simulink model "sixth_harmonic_report"  (R2013a)
settings: Solver=ode4  StartTime=0.0  StopTime=0.5  FixedStep=Ts  RelTol=1e-3
values from neighbouring files (symbols this model uses):
  Cdc = 200e-6    (= 0.0002)    [immd_design_elen.m]    (also in immd_efficiency.m = 5e-05; immd_simulation_base.m = 5e-05; sixth_harmonic_report.m = 0.003)
  Ldc = 1e-3    (= 0.001)    [sixth_harmonic_report.m]
  Lload = Xload/wout_fund    [acemp_sixth.m]    (also in immd_base_varyingmod.m = Xload/wout; immd_design_elen.m = Xload/wout; immd_efficiency.m = Xload/wout; immd_simulation_base.m = Xload/wout)
  Rload = Zload*pf    [acemp_sixth.m]    (also in immd_base_varyingmod.m; immd_design_elen.m; immd_efficiency.m; immd_simulation_base.m)
  Ts = 1e-6    (= 1e-06)    [acemp_sixth.m]    (also in immd_base_varyingmod.m = 1e-05; immd_design_elen.m; immd_efficiency.m; immd_simulation_base.m)
  Vsrms = 230    [sixth_harmonic_report.m]
libraries: powerlib x27, powerlib_meascontrol x27
settings Model: Creator=ugurm  LastModifiedBy=ugurm

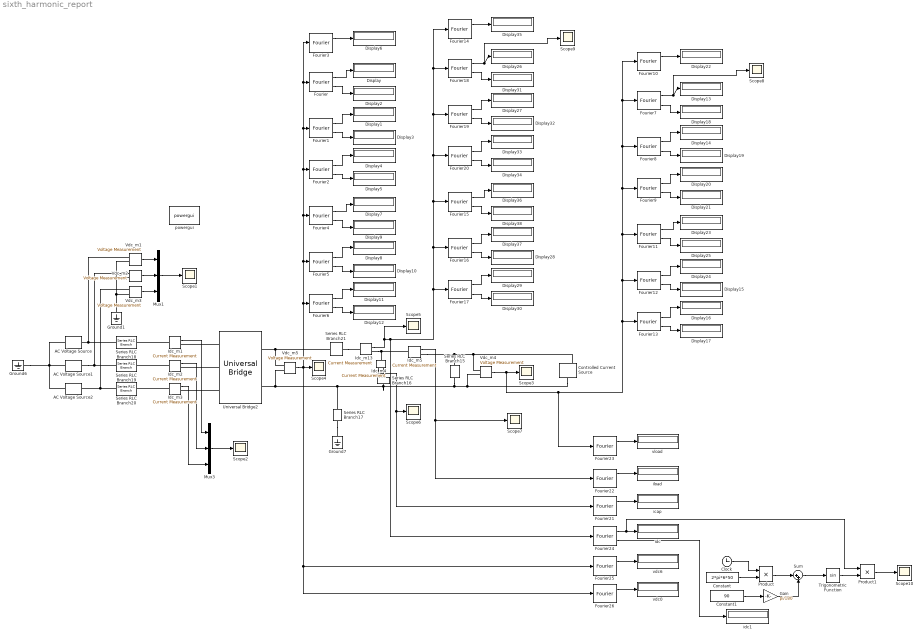
== system sixth_harmonic_report ==
  AC Voltage Source : powerlib/Electrical Sources/AC Voltage Source  Amplitude=Vsrms*sqrt(2)  Phase=0  Frequency=50  SampleTime=Ts  Measurements=None
  AC Voltage Source1 : powerlib/Electrical Sources/AC Voltage Source  Amplitude=Vsrms*sqrt(2)  Phase=-120  Frequency=50  SampleTime=Ts  Measurements=None
  AC Voltage Source2 : powerlib/Electrical Sources/AC Voltage Source  Amplitude=Vsrms*sqrt(2)  Phase=120  Frequency=50  SampleTime=Ts  Measurements=None
  Clock : Clock
  Constant : Constant  Value=2*pi*6*50
  Constant1 : Constant  Value=90
  Controlled Current Source : powerlib/Electrical Sources/Controlled Current Source  Initialize=on  Source_Type=AC  Amplitude=0  Phase=0  Frequency=0  Measurements=None
  Display{,1..38} (39 alike) : Display
  Fourier{,7,18,21..25} (8 alike) : powerlib_meascontrol/Measurements/Fourier  Freq=50  n=6  InInit=[0, 0]  Ts=0
  Fourier1 : powerlib_meascontrol/Measurements/Fourier  Freq=50  n=12  InInit=[0, 0]  Ts=0
  Fourier{3,10,14,26} (4 alike) : powerlib_meascontrol/Measurements/Fourier  Freq=50  n=0  InInit=[0, 0]  Ts=0
  Fourier11 : powerlib_meascontrol/Measurements/Fourier  Freq=50  n=24  InInit=[0, 0]  Ts=0
  Fourier12 : powerlib_meascontrol/Measurements/Fourier  Freq=50  n=30  InInit=[0, 0]  Ts=0
  Fourier13 : powerlib_meascontrol/Measurements/Fourier  Freq=50  n=36  InInit=[0, 0]  Ts=0
  Fourier15 : powerlib_meascontrol/Measurements/Fourier  Freq=50  n=24  InInit=[0, 0]  Ts=0
  Fourier16 : powerlib_meascontrol/Measurements/Fourier  Freq=50  n=30  InInit=[0, 0]  Ts=0
  Fourier17 : powerlib_meascontrol/Measurements/Fourier  Freq=50  n=36  InInit=[0, 0]  Ts=0
  Fourier19 : powerlib_meascontrol/Measurements/Fourier  Freq=50  n=12  InInit=[0, 0]  Ts=0
  Fourier2 : powerlib_meascontrol/Measurements/Fourier  Freq=50  n=18  InInit=[0, 0]  Ts=0
  Fourier20 : powerlib_meascontrol/Measurements/Fourier  Freq=50  n=18  InInit=[0, 0]  Ts=0
  Fourier4 : powerlib_meascontrol/Measurements/Fourier  Freq=50  n=24  InInit=[0, 0]  Ts=0
  Fourier5 : powerlib_meascontrol/Measurements/Fourier  Freq=50  n=30  InInit=[0, 0]  Ts=0
  Fourier6 : powerlib_meascontrol/Measurements/Fourier  Freq=50  n=36  InInit=[0, 0]  Ts=0
  Fourier8 : powerlib_meascontrol/Measurements/Fourier  Freq=50  n=12  InInit=[0, 0]  Ts=0
  Fourier9 : powerlib_meascontrol/Measurements/Fourier  Freq=50  n=18  InInit=[0, 0]  Ts=0
  Gain : Gain  Gain=pi/180
  Ground1 : powerlib/Elements/Ground  LConnTagsString=a
  Ground6 : powerlib/Elements/Ground  LConnTagsString=a
  Ground7 : powerlib/Elements/Ground  LConnTagsString=a
  Idc_m{1..5,13} (6 alike) : powerlib/Measurements/Current Measurement  PhasorSimulation=off  OutputType=Complex  PSBequivalent=0
  Mux1 : Mux  Inputs=3
  Mux3 : Mux  Inputs=3
  Product : Product
  Product1 : Product
  Scope{1..10} (10 alike) : Scope
      Scope1 settings: YMin=-1000  YMax=18000  SaveName=vabc
      Scope10 settings: YMin=-1  YMax=1  SaveName=iload1
      Scope2 settings: YMin=-1000  YMax=18000  SaveName=iabc
      Scope3 settings: YMin=-1000  YMax=18000  SaveName=vload
      Scope4 settings: YMin=-1000  YMax=18000  SaveName=vdc
      Scope5 settings: YMin=-1000  YMax=18000  SaveName=idc
      Scope6 settings: YMin=-1000  YMax=18000  SaveName=ic
      Scope7 settings: YMin=-1000  YMax=18000  SaveName=iload
      Scope8 settings: YMin=2.9  YMax=3.55  SaveName=vload1
      Scope9 settings: YMin=17.3  YMax=18.9  SaveName=vload2
  Series RLC Branch15 : powerlib/Elements/Series RLC Branch  LConnTagsString=__new0  RConnTagsString=__new0  BranchType=R  Resistance=Rload  Inductance=Lload  SetiL0=off  InitialCurrent=0  Capacitance=1e-6  Setx0=off  InitialVoltage=0  Measurements=None
  Series RLC Branch16 : powerlib/Elements/Series RLC Branch  LConnTagsString=__new0  RConnTagsString=__new0  BranchType=RC  Resistance=1e-9  Inductance=Lload  SetiL0=off  InitialCurrent=0  Capacitance=Cdc  Setx0=off  InitialVoltage=0  Measurements=None
  Series RLC Branch17 : powerlib/Elements/Series RLC Branch  LConnTagsString=__new0  RConnTagsString=__new0  BranchType=R  Resistance=1e12  Inductance=Lload  SetiL0=off  InitialCurrent=0  Capacitance=1e-6  Setx0=off  InitialVoltage=0  Measurements=None
  Series RLC Branch18 : powerlib/Elements/Series RLC Branch  LConnTagsString=__new0  RConnTagsString=__new0  BranchType=RL  Resistance=1e-6  Inductance=1e-9  SetiL0=off  InitialCurrent=0  Capacitance=100e-6  Setx0=off  InitialVoltage=0  Measurements=None
  Series RLC Branch19 : powerlib/Elements/Series RLC Branch  LConnTagsString=__new0  RConnTagsString=__new0  BranchType=RL  Resistance=1e-6  Inductance=1e-9  SetiL0=off  InitialCurrent=0  Capacitance=100e-6  Setx0=off  InitialVoltage=0  Measurements=None
  Series RLC Branch20 : powerlib/Elements/Series RLC Branch  LConnTagsString=__new0  RConnTagsString=__new0  BranchType=RL  Resistance=1e-6  Inductance=1e-9  SetiL0=off  InitialCurrent=0  Capacitance=100e-6  Setx0=off  InitialVoltage=0  Measurements=None
  Series RLC Branch21 : powerlib/Elements/Series RLC Branch  LConnTagsString=__new0  RConnTagsString=__new0  BranchType=RL  Resistance=1e-6  Inductance=Ldc  SetiL0=off  InitialCurrent=0  Capacitance=100e-6  Setx0=off  InitialVoltage=0  Measurements=None
  Sum : Sum  Inputs=|++
  Trigonometric Function : Trigonometry
  Universal Bridge2 : powerlib/Power Electronics/Universal Bridge  Arms=3  SnubberResistance=1e5  SnubberCapacitance=inf  Device=Diodes  Ron=1e-6  Lon=0  ForwardVoltages="[  0  0  ]"  ForwardVoltage=0  GTOparameters=[ 10e-6 , 20e-6 ]  IGBTparameters=[0,0]  Measurements=None  Measurements_2=None  converterType=Rectifier
  Vdc_m{1..5} (5 alike) : powerlib/Measurements/Voltage Measurement  PhasorSimulation=off  OutputType=Complex  PSBequivalent=0
  icap : Display
  idc : Display
  idc1 : Display
  iload : Display
  powergui : powerlib/powergui  Priority=1  SimulationMode=Discrete  SolverType=Tustin  SampleTime=Ts  frequency=60  SPID=off  DisableSnubberDevices=off  DisableRonSwitches=off  DisableVfSwitches=off  SwTol=0  Interpol=off  DisplayEquations=off  frequencyindice=0  Pbase=100e6  ErrMax=1e-4  Iterations=50  UnitsV=kV  UnitsW=MW  FunctionMessages=off  echomessages=off  HookPort=off  EnableUseOfTLC=off  x0status=blocks  RestoreLinks=warning  ResistiveCurrentMeasurement=off  Frange=[0:2:500]  Ylog=off  Xlog=on  ShowGrid=off  save=off  variable=ZData  structure=vdc  ZoomFFT=off  StartTime=0.1  cycles=10  DisplayStyle=6  fundamental=50  FreqAxis=off  MaxFrequency=1000  frequencyindicesteady=1  RmsSteady=1  display=off  Ts=0  methode=off
  vdc0 : Display
  vdc6 : Display
  vload : Display
  wires:
  Vdc_m1/1 -> Mux1/1
  Vdc_m2/1 -> Mux1/2
  Vdc_m3/1 -> Mux1/3
  Mux1/1 -> Scope1/1
  Mux3/1 -> Scope2/1
  Idc_m1/1 -> Mux3/1
  Idc_m2/1 -> Mux3/2
  Idc_m3/1 -> Mux3/3
  Fourier/1 -> Display/1
  Fourier1/1 -> Display1/1
  Fourier/2 -> Display2/1
  Fourier1/2 -> Display3/1
  Fourier2/1 -> Display4/1
  Fourier2/2 -> Display5/1
  Fourier3/1 -> Display6/1
  Fourier4/1 -> Display7/1
  Fourier5/1 -> Display8/1
  Fourier4/2 -> Display9/1
  Fourier5/2 -> Display10/1
  Fourier6/1 -> Display11/1
  Fourier6/2 -> Display12/1
  Vdc_m4/1 -> Scope3/1, Fourier23/1, Fourier12/1, Fourier11/1, Fourier10/1, Fourier7/1, Fourier8/1, Fourier9/1, Fourier13/1
  Fourier7/1 -> Scope8/1, Display13/1
  Fourier8/1 -> Display14/1
  Fourier7/2 -> Display18/1
  Fourier8/2 -> Display19/1
  Fourier9/1 -> Display20/1
  Fourier9/2 -> Display21/1
  Fourier10/1 -> Display22/1
  Fourier11/1 -> Display23/1
  Fourier12/1 -> Display24/1
  Fourier11/2 -> Display25/1
  Fourier12/2 -> Display15/1
  Fourier13/1 -> Display16/1
  Fourier13/2 -> Display17/1
  Fourier18/1 -> Scope9/1, Display26/1
  Fourier19/1 -> Display27/1
  Fourier18/2 -> Display31/1
  Fourier19/2 -> Display32/1
  Fourier20/1 -> Display33/1
  Fourier20/2 -> Display34/1
  Fourier14/1 -> Display35/1
  Fourier15/1 -> Display36/1
  Fourier16/1 -> Display37/1
  Fourier15/2 -> Display38/1
  Fourier16/2 -> Display28/1
  Fourier17/1 -> Display29/1
  Fourier17/2 -> Display30/1
  Idc_m5/1 -> Fourier22/1, Scope7/1
  Idc_m4/1 -> Fourier21/1, Scope6/1
  Fourier21/1 -> icap/1
  Fourier22/1 -> iload/1
  Fourier23/1 -> vload/1
  Idc_m13/1 -> Fourier24/1, Fourier16/1, Fourier15/1, Fourier14/1, Fourier18/1, Fourier19/1, Fourier20/1, Fourier17/1, Scope5/1
  Vdc_m5/1 -> Fourier6/1, Fourier5/1, Fourier4/1, Fourier2/1, Fourier1/1, Fourier3/1, Fourier/1, Fourier26/1, Fourier25/1, Scope4/1
  Fourier25/1 -> vdc6/1
  Fourier26/1 -> vdc0/1
  Fourier24/2 -> idc1/1
  Clock/1 -> Product/1
  Constant/1 -> Product/2
  Product/1 -> Sum/1
  Gain/1 -> Sum/2
  Constant1/1 -> Gain/1
  Sum/1 -> Trigonometric Function/1
  Trigonometric Function/1 -> Product1/2
  Product1/1 -> Scope10/1
  Fourier24/1 -> Product1/1, idc/1
  connections:
  Vdc_m4/LConn1 -- Controlled Current Source/LConn1 -- Series RLC Branch15/RConn1 -- Idc_m5/RConn1
  Vdc_m4/LConn2 -- Controlled Current Source/RConn1 -- Series RLC Branch17/LConn1 -- Vdc_m5/LConn2 -- Universal Bridge2/RConn2 -- Series RLC Branch16/RConn1 -- Series RLC Branch15/LConn1
  Series RLC Branch17/RConn1 -- Ground7/LConn1
  Series RLC Branch20/RConn1 -- Vdc_m3/LConn1 -- AC Voltage Source2/RConn1
  AC Voltage Source1/RConn1 -- Vdc_m2/LConn1 -- Series RLC Branch19/RConn1
  Series RLC Branch18/RConn1 -- Vdc_m1/LConn1 -- AC Voltage Source/RConn1
  Series RLC Branch21/LConn1 -- Idc_m13/LConn1
  Series RLC Branch21/RConn1 -- Vdc_m5/LConn1 -- Universal Bridge2/RConn1
  AC Voltage Source1/LConn1 -- Ground6/LConn1 -- AC Voltage Source/LConn1 -- AC Voltage Source2/LConn1
  Idc_m1/LConn1 -- Series RLC Branch18/LConn1
  Idc_m2/LConn1 -- Series RLC Branch19/LConn1
  Idc_m3/LConn1 -- Series RLC Branch20/LConn1
  Ground1/LConn1 -- Vdc_m3/LConn2 -- Vdc_m1/LConn2 -- Vdc_m2/LConn2
  Universal Bridge2/LConn1 -- Idc_m1/RConn1
  Universal Bridge2/LConn2 -- Idc_m2/RConn1
  Universal Bridge2/LConn3 -- Idc_m3/RConn1
  Idc_m4/RConn1 -- Series RLC Branch16/LConn1
  Idc_m13/RConn1 -- Idc_m5/LConn1 -- Idc_m4/LConn1
